simulink model "M_M_1_model"  (R2021a)
settings: Solver=VariableStepAuto  StartTime=0.0  StopTime=10.0  RelTol=1e-3
undefined symbols (not defined in the file): m, n
settings Model: Creator=mluser  LastModifiedBy=mluser

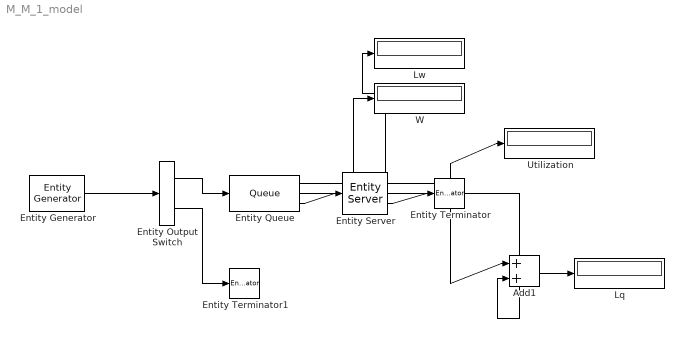
== system M_M_1_model ==
  Add1 : Sum
  Entity Output Switch : EntityOutputSwitch  InputPortMessageModes=m  OutputPortMessageModes=m,m  SwitchAttributeName=Attribute1
  Entity Generator : EntityGenerator  OutputPortMessageModes=m  TimeSource=MATLAB action  IntergenerationTimeAction=|  EntityType=Structured  EntityTypeName=Entity
      | dt = rand(1,1);
      | persistent rngInit;
      | if isempty(rngInit)
      |     seed = 12345;
      |     rng(seed);
      |     rngInit = true;
      | end
      | 
      | % Pattern: Exponential distribution
      | mu = 0.1;
      | dt = -mu * log(1 - rand());
  Entity Queue : Queue  InputPortMessageModes=m  OutputPortMessageModes=n,n,m  Capacity=inf  AverageWait=on  AverageQueueLength=on
      settings: OutputPortMap=o2,o3,o5
  Entity Server : EntityServer  InputPortMessageModes=m  OutputPortMessageModes=n,m  Capacity=1  Utilization=on
      settings: OutputPortMap=o5,o9
  Entity Terminator : EntityTerminator  InputPortMessageModes=m
  Entity Terminator1 : EntityTerminator  InputPortMessageModes=m
  Lq : Display
  Lw : Display
  Utilization : Display
  W : Display
  wires:
  Entity Server/2 -> Entity Terminator/1
  Entity Queue/3 -> Entity Server/1
  Entity Generator/1 -> Entity Output Switch/1
  Entity Output Switch/1 -> Entity Queue/1
  Entity Output Switch/2 -> Entity Terminator1/1
  Entity Queue/2 -> Add1/2, Lw/1
  Entity Queue/1 -> W/1
  Entity Server/1 -> Utilization/1, Add1/1
  Add1/1 -> Lq/1
